simulink model "consensus_CHECKED"  (Simulink 8.0)
settings: Solver=ode45  StartTime=0.0  StopTime=10.0  RelTol=1e-3
settings Model: Creator=chepeadan  LastModifiedBy=koehler
settings DataIOCC: SignalLoggingSaveFormat=ModelDataLogs
settings DebuggingCC: FcnCallInpInsideContextMsg=UseLocalSettings  StrictBusMsg=Warning
settings GRTTargetCC: CombineOutputUpdateFcns=off  GRTInterface=on

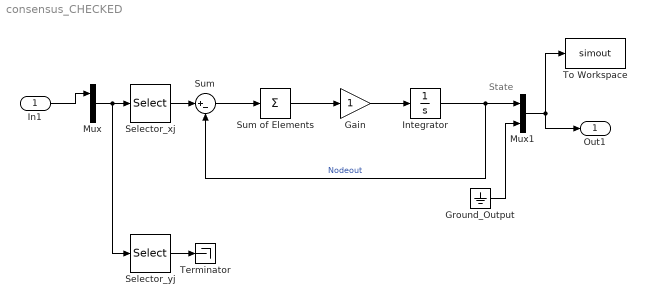
== system consensus_CHECKED ==
  note: State
  In1 : Inport
  Gain : Gain
  Ground_Output : Ground
  Integrator : Integrator  InitialCondition=100*(rand()-0.5)
  Mux : Mux  Inputs=2
  Mux1 : Mux  Inputs=2
  Selector_xj : Selector  InputPortWidth=2  IndexOptions=Index vector (dialog)  Indices=[1]  OutputSizes=1
  Selector_yj : Selector  InputPortWidth=2  IndexOptions=Index vector (dialog)  Indices=[1]  OutputSizes=1
  Sum : Sum  Inputs=|+-
  Sum of Elements : Sum  Inputs=+
  Terminator : Terminator
  To Workspace : ToWorkspace  VariableName=simout  SampleTime=-1  SaveFormat=Structure With Time
  Out1 : Outport
  wires:
  In1/1 -> Mux/1
  Sum/1 -> Sum of Elements/1
  Sum of Elements/1 -> Gain/1
  Gain/1 -> Integrator/1
  Integrator/1 -> Mux1/1, Sum/2  "Nodeout"
  Selector_xj/1 -> Sum/1
  Mux/1 -> Selector_yj/1, Selector_xj/1
  Selector_yj/1 -> Terminator/1
  Mux1/1 -> Out1/1, To Workspace/1
  Ground_Output/1 -> Mux1/2
